simulink model "asgers_sim"  (R2017b)
settings: Solver=VariableStepAuto  StartTime=0.0  StopTime=2  RelTol=1e-3
values from neighbouring files (symbols this model uses):
  alpha = 0.1    [Asgers.m]
  Kp = 1/M    [Asgers.m]
  tau_d = 1/(omega_c*sqrt(alpha))    [Asgers.m]
  tau_i = Ni/omega_c    (= 0.104166666667)    [Asgers.m]
settings Model: Creator=asger  LastModifiedBy=asger

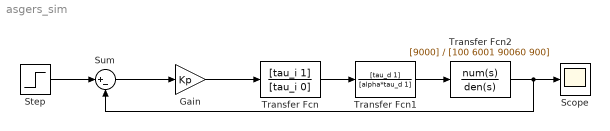
== system asgers_sim ==
  Gain : Gain  Gain=Kp
  Scope : Scope
  Step : Step  Time=0  SampleTime=0
  Sum : Sum  Inputs=|+-
  Transfer Fcn : TransferFcn  Numerator=[tau_i 1]  Denominator=[tau_i 0]
  Transfer Fcn1 : TransferFcn  Numerator=[tau_d 1]  Denominator=[alpha*tau_d 1]
  Transfer Fcn2 : TransferFcn  Numerator=[9000]  Denominator=[100 6001 90060 900]
  wires:
  Step/1 -> Sum/1
  Sum/1 -> Gain/1
  Gain/1 -> Transfer Fcn/1
  Transfer Fcn/1 -> Transfer Fcn1/1
  Transfer Fcn1/1 -> Transfer Fcn2/1
  Transfer Fcn2/1 -> Sum/2, Scope/1
